simulink model "ACC_Sensor"  (R2025b)
settings: Solver=VariableStepAuto  StartTime=0.0  StopTime=10.0  RelTol=1e-3
libraries: simulink x2
settings Model: Creator=ghazal  LastModifiedBy=ghazal

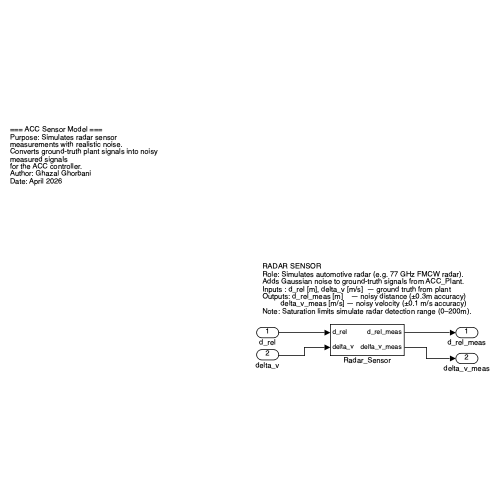
[thumbnail: Simulink's stored preview of the top-level diagram]
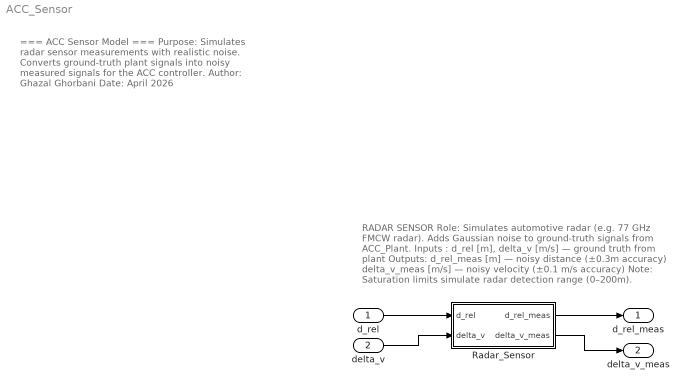
== system ACC_Sensor ==
  note: RADAR SENSOR
      | Role: Simulates automotive radar (e.g. 77 GHz FMCW radar).
      | Adds Gaussian noise to ground-truth signals from ACC_Plant.
      | Inputs : d_rel [m], delta_v [m/s]  — ground truth from plant
      | Outputs: d_rel_meas [m]    — noisy distance (±0.3m accuracy)
      |          delta_v_meas [m/s] — noisy velocity (±0.1 m/s accuracy)
      | Note: Saturation limits simulate radar detection range (0–200m).
  note: === ACC Sensor Model ===
      | Purpose: Simulates radar sensor measurements with realistic noise.
      | Converts ground-truth plant signals into noisy measured signals
      | for the ACC controller.
      | Author: Ghazal Ghorbani
      | Date: April 2026
  d_rel : Inport
  delta_v : Inport  Port=2
  Radar_Sensor : Subsystem
  d_rel_meas : Outport
  delta_v_meas : Outport  Port=2
  wires:
  Radar_Sensor/1(d_rel_meas) -> d_rel_meas/1
  Radar_Sensor/2(delta_v_meas) -> delta_v_meas/1
  d_rel/1 -> Radar_Sensor/1(d_rel)
  delta_v/1 -> Radar_Sensor/2(delta_v)

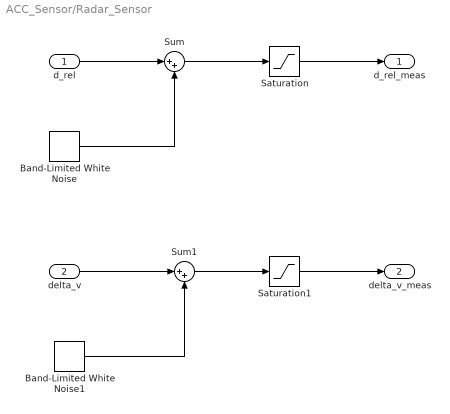
== system ACC_Sensor/Radar_Sensor ==
  d_rel : Inport
  delta_v : Inport  Port=2
  Band-Limited White Noise : simulink/Sources/Band-Limited White Noise  Cov=[0.0009]  Ts=0.01  seed=[23341]
  Band-Limited White Noise1 : simulink/Sources/Band-Limited White Noise  Cov=[0.01]  Ts=0.01  seed=[23342]
  Saturation : Saturate  UpperLimit=200  LowerLimit=0
  Saturation1 : Saturate  UpperLimit=50  LowerLimit=-50
  Sum : Sum  Inputs=|++
  Sum1 : Sum  Inputs=|++
  d_rel_meas : Outport
  delta_v_meas : Outport  Port=2
  wires:
  d_rel/1 -> Sum/1
  Sum/1 -> Saturation/1
  Band-Limited White Noise/1 -> Sum/2
  Saturation/1 -> d_rel_meas/1
  delta_v/1 -> Sum1/1
  Band-Limited White Noise1/1 -> Sum1/2
  Sum1/1 -> Saturation1/1
  Saturation1/1 -> delta_v_meas/1
